simulink model "ksrbl_4k4t_hdtrig"  (Simulink 6.2)
settings: Solver=ode45  StartTime=0.0  StopTime=20000  RelTol=1e-3
libraries: xbsIndex_r3 x1214, casper_library x120, xps_library x20
(part 7 of 26)

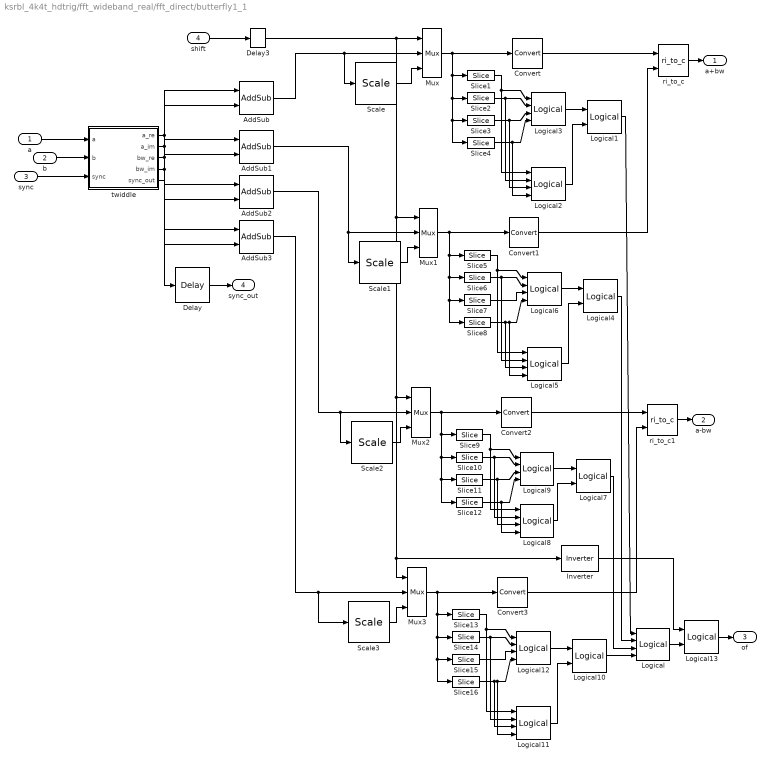
== system ksrbl_4k4t_hdtrig/fft_wideband_real/fft_direct/butterfly1_1 ==
  a : Inport  Port=1  LatchInput=off
  b : Inport  Port=2  LatchInput=off
  sync : Inport  Port=3  LatchInput=off
  shift : Inport  Port=4  LatchInput=off
  AddSub : xbsIndex_r3/AddSub  mode=Addition  precision=Full  arith_type=Unsigned  n_bits=8  bin_pt=2  quantization=Truncate  overflow=Wrap  latency=add_latency  explicit_period=off  period=1  use_carryin=off  use_carryout=off  en=off  dbl_ovrd=off  show_param=on  use_core=on  pipeline=on  use_rpm=on  gen_core=on
      settings: xl_area=[0, 0, 0, 0, 0, 0, 0]
  AddSub1 : xbsIndex_r3/AddSub  mode=Addition  precision=Full  arith_type=Unsigned  n_bits=8  bin_pt=2  quantization=Truncate  overflow=Wrap  latency=add_latency  explicit_period=off  period=1  use_carryin=off  use_carryout=off  en=off  dbl_ovrd=off  show_param=on  use_core=on  pipeline=on  use_rpm=on  gen_core=on
      settings: xl_area=[0, 0, 0, 0, 0, 0, 0]
  AddSub2 : xbsIndex_r3/AddSub  mode=Subtraction  precision=Full  arith_type=Unsigned  n_bits=8  bin_pt=2  quantization=Truncate  overflow=Wrap  latency=add_latency  explicit_period=off  period=1  use_carryin=off  use_carryout=off  en=off  dbl_ovrd=off  show_param=on  use_core=on  pipeline=on  use_rpm=on  gen_core=on
      settings: xl_area=[0, 0, 0, 0, 0, 0, 0]
  AddSub3 : xbsIndex_r3/AddSub  mode=Subtraction  precision=Full  arith_type=Unsigned  n_bits=8  bin_pt=2  quantization=Truncate  overflow=Wrap  latency=add_latency  explicit_period=off  period=1  use_carryin=off  use_carryout=off  en=off  dbl_ovrd=off  show_param=on  use_core=on  pipeline=on  use_rpm=on  gen_core=on
      settings: xl_area=[0, 0, 0, 0, 0, 0, 0]
  Convert{,1..3} (4 alike) : xbsIndex_r3/Convert  arith_type="Signed  (2's comp)"  n_bits=BitWidth  bin_pt=BitWidth-1  quantization=Truncate  overflow=Wrap  latency=add_latency  explicit_period=off  period=1  dbl_ovrd=off  show_param=off  inserted_by_tool=off  pipeline=off
      settings: xl_area=[0, 0, 0, 0, 0, 0, 0]
  Delay : xbsIndex_r3/Delay  latency=2 * add_latency + 1  reg_retiming=off  explicit_period=off  period=1  en=off  accept_only_valid=off  init_zero=on  dbl_ovrd=off  show_param=off
      settings: xl_area=[0, 0, 0, 0, 0, 0, 0]
  Delay3 : xbsIndex_r3/Delay  latency=1  reg_retiming=off  explicit_period=off  period=1  en=off  accept_only_valid=off  init_zero=on  dbl_ovrd=off  show_param=off
      settings: xl_area=[0, 0, 0, 0, 0, 0, 0]
  Inverter : xbsIndex_r3/Inverter  latency=0  explicit_period=off  period=1  en=off  dbl_ovrd=off  show_param=off
      settings: xl_area=[0, 0, 0, 0, 0, 0, 0]
  Logical : xbsIndex_r3/Logical  logical_function=OR  inputs=4  precision=Full  arith_type=Unsigned  n_bits=8  bin_pt=2  align_bp=on  latency=1  explicit_period=off  period=1  en=off  dbl_ovrd=off  show_param=off
      settings: xl_area=[0, 0, 0, 0, 0, 0, 0]
  Logical{1,4,7,10} (4 alike) : xbsIndex_r3/Logical  logical_function=OR  inputs=2  precision=Full  arith_type=Unsigned  n_bits=8  bin_pt=2  align_bp=off  latency=1  explicit_period=off  period=1  en=off  dbl_ovrd=off  show_param=off
      settings: xl_area=[0, 0, 0, 0, 0, 0, 0]
  Logical{2,5,8,11} (4 alike) : xbsIndex_r3/Logical  logical_function=NOR  inputs=4  precision=Full  arith_type=Unsigned  n_bits=8  bin_pt=2  align_bp=off  latency=1  explicit_period=off  period=1  en=off  dbl_ovrd=off  show_param=off
      settings: xl_area=[0, 0, 0, 0, 0, 0, 0]
  Logical{3,6,9,12} (4 alike) : xbsIndex_r3/Logical  logical_function=AND  inputs=4  precision=Full  arith_type=Unsigned  n_bits=8  bin_pt=2  align_bp=off  latency=1  explicit_period=off  period=1  en=off  dbl_ovrd=off  show_param=off
      settings: xl_area=[0, 0, 0, 0, 0, 0, 0]
  Logical13 : xbsIndex_r3/Logical  logical_function=AND  inputs=2  precision=Full  arith_type=Unsigned  n_bits=8  bin_pt=2  align_bp=off  latency=1  explicit_period=off  period=1  en=off  dbl_ovrd=off  show_param=off
      settings: xl_area=[0, 0, 0, 0, 0, 0, 0]
  Mux{,1..3} (4 alike) : xbsIndex_r3/Mux  inputs=2  precision=Full  arith_type="Signed  (2's comp)"  n_bits=8  bin_pt=2  quantization=Truncate  overflow=Wrap  latency=1  explicit_period=off  period=1  en=off  dbl_ovrd=off  show_param=off  mux_type=off  use_rpm=off  gen_core=off
      settings: xl_area=[0, 0, 0, 0, 0, 0, 0]
  Scale{,1..3} (4 alike) : xbsIndex_r3/Scale  scale_factor=-1  explicit_period=off  period=1  dbl_ovrd=off
  Slice{1,5,9,13} (4 alike) : xbsIndex_r3/Slice  mode=Upper Bit Location + Width  nbits=1  bit1=0  base1=MSB of Input  bit0=0  base0=LSB of Input  boolean_output=on  explicit_period=off  period=1  dbl_ovrd=off
  Slice{2,6,10,14} (4 alike) : xbsIndex_r3/Slice  mode=Upper Bit Location + Width  nbits=1  bit1=-1  base1=MSB of Input  bit0=0  base0=LSB of Input  boolean_output=on  explicit_period=off  period=1  dbl_ovrd=off
  Slice{3,7,11,15} (4 alike) : xbsIndex_r3/Slice  mode=Upper Bit Location + Width  nbits=1  bit1=-2  base1=MSB of Input  bit0=0  base0=LSB of Input  boolean_output=on  explicit_period=off  period=1  dbl_ovrd=off
  Slice{4,8,12,16} (4 alike) : xbsIndex_r3/Slice  mode=Upper Bit Location + Width  nbits=1  bit1=-3  base1=MSB of Input  bit0=0  base0=LSB of Input  boolean_output=on  explicit_period=off  period=1  dbl_ovrd=off
  ri_to_c : casper_library/Misc/ri_to_c
  ri_to_c1 : casper_library/Misc/ri_to_c
  twiddle : Subsystem  BlockChoice=twiddle_general_3mult
      link override twiddle_general_3mult: Coeffs="[1+0i                     1-0.003068i        0.99998-0.0061359i       0.99996-0.0092038i       0.99992-0.012272i        0.99988-0.015339i        0.99983-0.018407i        0.99977-0.021474i         0.9997-0.024541i        0.99962-0.027608i        0.99953-0.030675i        0.99943-0.033741i        0.99932-0.036807i         0.9992-0.039873i        0.99908-0.042938i        0.99894-0.046003i         0.9988-0.049068i        0.99864-0.052132i        0.99848-0.055195i         0.9983-0.058258i        0.99812-0.061321i        0.99793-0.064383i        0.99772-0.067444i        0.99751-0.070505i        0.99729-0.073565i        0.99706-0.076624i        0.99682-0.079682i        0.99657-0.08274i         0.99631-0.085797i        0.99604-0.088854i        0.99577-0.091909i        0.99548-0.094963i        0.99518-0.098017i        0.99488-0.10107i         0.99456-0.10412i         0.99424-0.10717i         0.99391-0.11022i         0.99356-0.11327i         0.99321-0.11632i         0.99285-0.11937i         0.99248-0.12241i          0.9921-0.12545i         0.99171-0.1285i          0.99131-0.13154i          0.9909-0.13458i         0.99049-0.13762i         0.99006-0.14066i         0.98962-0.1437i          0.98918-0.14673i         0.98872-0.14976i         0.98826-0.1528i          0.98778-0.15583i          0.9873-0.15886i         0.98681-0.16189i         0.98631-0.16491i          0.9858-0.16794i         0.98528-0.17096i         0.98475-0.17398i         0.98421-0.177i           0.98366-0.18002i         0.98311-0.18304i         0.98254-0.18606i         0.98196-0.18907i         0.98138-0.19208i         0.98079-0.19509i         0.98018-0.1981i          0.97957-0.2011i          0.97895-0.20411i         0.97832-0.20711i         0.97768-0.21011i         0.97703-0.21311i         0.97637-0.21611i          0.9757-0.2191i          0.97503-0.22209i         0.97434-0.22508i         0.97364-0.22807i         0.97294-0.23106i         0.97223-0.23404i          0.9715-0.23702i         0.97077-0.24i            0.97003-0.24298i         0.96928-0.24596i         0.96852-0.24893i         0.96775-0.2519i          0.96698-0.25487i         0.96619-0.25783i         0.96539-0.26079i         0.96459-0.26375i         0.96378-0.26671i         0.96295-0.26967i         0.96212-0.27262i         0.96128-0.27557i         0.96043-0.27852i         0.95957-0.28146i          0.9587-0.28441i         0.95783-0.28735i         0.95694-0.29028i         0.95605-0.29322i         0.95514-0.29615i         0.95423-0.29908i         0.95331-0.30201i         0.95238-0.30493i         0.95144-0.30785i         0.95049-0.31077i         0.94953-0.31368i         0.94856-0.31659i         0.94759-0.3195i           0.9466-0.32241i         0.94561-0.32531i          0.9446-0.32821i         0.94359-0.33111i         0.94257-0.334i           0.94154-0.33689i         0.94051-0.33978i         0.93946-0.34266i          0.9384-0.34554i         0.93734-0.34842i         0.93627-0.35129i         0.93518-0.35416i         0.93409-0.35703i         0.93299-0.3599i          0.93188-0.36276i         0.93077-0.36561i         0.92964-0.36847i         0.92851-0.37132i         0.92736-0.37416i         0.92621-0.37701i         0.92505-0.37985i         0.92388-0.38268i          0.9227-0.38552i         0.92151-0.38835i         0.92032-0.39117i         0.91911-0.39399i          0.9179-0.39681i         0.91668-0.39962i         0.91545-0.40243i         0.91421-0.40524i         0.91296-0.40804i         0.91171-0.41084i         0.91044-0.41364i         0.90917-0.41643i         0.90789-0.41922i          0.9066-0.422i            0.9053-0.42478i         0.90399-0.42756i         0.90267-0.43033i         0.90135-0.43309i         0.90002-0.43586i         0.89867-0.43862i         0.89732-0.44137i         0.89597-0.44412i          0.8946-0.44687i         0.89322-0.44961i         0.89184-0.45235i         0.89045-0.45508i         0.88905-0.45781i         0.88764-0.46054i         0.88622-0.46326i          0.8848-0.46598i         0.88336-0.46869i ...(+21593 chars)   ]"  StepPeriod=0  BitWidth=18  add_latency=4  mult_latency=6  bram_latency=4
      link override twiddle_general_3mult/coeff_gen: BlockChoice=br_coeff_gen
      link override twiddle_general_3mult/coeff_gen/br_coeff_gen: Coeffs=[1 2 3 4 5 6 7]  StepPeriod=4  BitWidth=10  bram_latency=6
      link override twiddle_general_3mult/coeff_gen/br_coeff_gen/ROM: distributed_mem=off
      link override twiddle_general_3mult/coeff_gen/br_coeff_gen/ROM1: distributed_mem=off
      link override twiddle_general_3mult/coeff_gen/static_coeff_gen/Constant: equ=P=C
      link override twiddle_general_3mult/coeff_gen/static_coeff_gen/Constant1: equ=P=C
      settings: AttributesFormatString=%<BlockChoice>  TemplateBlock=casper_library/FFTs/Twiddle/twiddle  MemberBlocks=twiddle_coeff_0,twiddle_coeff_1,twiddle_general_3mult,twiddle_general_4mult,twiddle_stage_2
  a+bw : Outport
  a-bw : Outport  Port=2
  of : Outport  Port=3
  sync_out : Outport  Port=4
  wires:
  Inverter/1 -> Logical13/1
  Logical13/1 -> of/1
  Logical/1 -> Logical13/2
  Delay3/1 -> Inverter/1, Mux3/1, Mux2/1, Mux1/1, Mux/1
  Logical7/1 -> Logical/3
  AddSub3/1 -> Scale3/1, Mux3/2
  Logical10/1 -> Logical/4
  Logical11/1 -> Logical10/2
  Logical12/1 -> Logical10/1
  Slice16/1 -> Logical11/3, Logical11/4, Logical12/4
  Slice15/1 -> Logical12/3
  Slice14/1 -> Logical11/2, Logical12/2
  Slice13/1 -> Logical11/1, Logical12/1
  Convert3/1 -> ri_to_c1/2
  Scale3/1 -> Mux3/3
  Mux3/1 -> Slice16/1, Slice15/1, Slice14/1, Slice13/1, Convert3/1
  AddSub2/1 -> Scale2/1, Mux2/2
  Logical8/1 -> Logical7/2
  Logical9/1 -> Logical7/1
  Slice12/1 -> Logical8/4, Logical9/4
  Slice11/1 -> Logical8/3, Logical9/3
  Slice10/1 -> Logical8/2, Logical9/2
  Slice9/1 -> Logical8/1, Logical9/1
  Convert2/1 -> ri_to_c1/1
  Scale2/1 -> Mux2/3
  Mux2/1 -> Slice12/1, Slice11/1, Slice10/1, Slice9/1, Convert2/1
  Logical4/1 -> Logical/2
  Logical5/1 -> Logical4/2
  Logical6/1 -> Logical4/1
  Slice8/1 -> Logical5/3, Logical5/4, Logical6/4
  Slice7/1 -> Logical6/3
  Slice6/1 -> Logical5/2, Logical6/2
  Slice5/1 -> Logical5/1, Logical6/1
  Convert1/1 -> ri_to_c/2
  Scale1/1 -> Mux1/3
  Mux1/1 -> Slice8/1, Slice7/1, Slice6/1, Slice5/1, Convert1/1
  Logical1/1 -> Logical/1
  Logical2/1 -> Logical1/2
  Logical3/1 -> Logical1/1
  Slice4/1 -> Logical2/4, Logical3/4
  Slice3/1 -> Logical2/3, Logical3/3
  Slice2/1 -> Logical2/2, Logical3/2
  Slice1/1 -> Logical2/1, Logical3/1
  Convert/1 -> ri_to_c/1
  Scale/1 -> Mux/3
  Mux/1 -> Slice4/1, Slice3/1, Slice2/1, Slice1/1, Convert/1
  shift/1 -> Delay3/1
  AddSub1/1 -> Scale1/1, Mux1/2
  AddSub/1 -> Scale/1, Mux/2
  Delay/1 -> sync_out/1
  ri_to_c1/1 -> a-bw/1
  ri_to_c/1 -> a+bw/1
  a/1 -> twiddle/1(a)
  b/1 -> twiddle/2(b)
  sync/1 -> twiddle/3(sync)
  twiddle/1(a_re) -> AddSub/1, AddSub2/1
  twiddle/2(a_im) -> AddSub1/1, AddSub3/1
  twiddle/3(bw_re) -> AddSub/2, AddSub2/2
  twiddle/4(bw_im) -> AddSub1/2, AddSub3/2
  twiddle/5(sync_out) -> Delay/1
